simulink model "cubli_XYZ_extensive_simulations"  (R2016a)
settings: Solver=VariableStepAuto  StartTime=0.0  StopTime=10  FixedStep=0.001  RelTol=1e-3
values from neighbouring files (symbols this model uses):
  a = 0.15    [init.m]
  M = 2.5    [init.m]    (also in skew.m = [0 -z y)
  m = 0.204    [init.m]
  s = size(delta_i)    [accessibility_test.m]    (also in observability_test.m = size(delta_i,1))
  state0 = get_equilibrium(0, -pi/4, pi/2, f, state)    [init.m]
undefined symbols (not defined in the file or in its folder): X, Y, Z
libraries: sm_lib x15, nesl_utility x13
(part 6 of 9)

== matlab function cubli_XYZ_extensive_simulations/Cubli/Reference/slerp input ==
  data: R0 output; Rf output; t output; th output; time input; state0 parameter; final_time parameter; theta parameter
function [R0, Rf, t, th] = slerp_input(time, state0, final_time, theta)
 
th = theta * pi / 180;

t = time / final_time;
deltaR = rotz(th);

R0 = rotx(state0(1))*roty(state0(2))*rotz(state0(3));
Rf = deltaR * R0;

if time >= final_time
    t = 1;
%     Rf = rotx(state0(1))*roty(state0(2))*rotz(state0(3));
%     R0 = deltaR * Rf;
%     t = (time - duration) / duration;
end

% if time >= 2 * duration
%     t = 1;
% end
